simulink model "Tire1_basic02"  (R2022a)
settings: Solver=VariableStepAuto  StartTime=0.0  StopTime=100  RelTol=1e-3
undefined symbols (not defined in the file or in its folder): Mass
libraries: nesl_utility x2, fl_lib x1, sdl_lib x1
settings Model: Creator=amyyang  LastModifiedBy=amyyang
settings SolverCC: AlgebraicLoopSolver=TrustRegion
settings DebuggingCC: UnconnectedInputMsg=warning  UnconnectedOutputMsg=warning  UnconnectedLineMsg=warning  SFMachineParentedDataDiag=warning
settings RTWCC: DLArmComputeVersion=19.05
settings SimscapeCC: SimscapeLogType=local  SimscapeLogToSDI=on  SimscapeLogLimitData=off

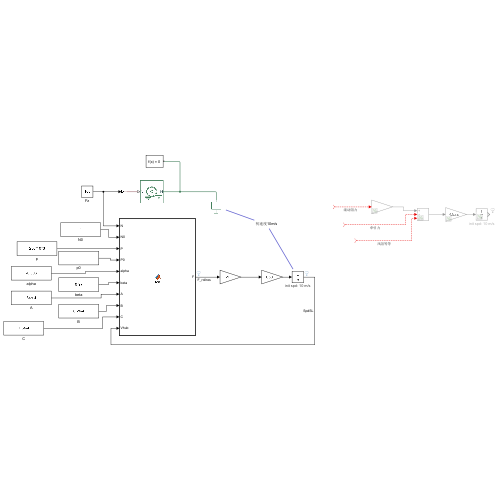
[thumbnail: Simulink's stored preview of the top-level diagram]
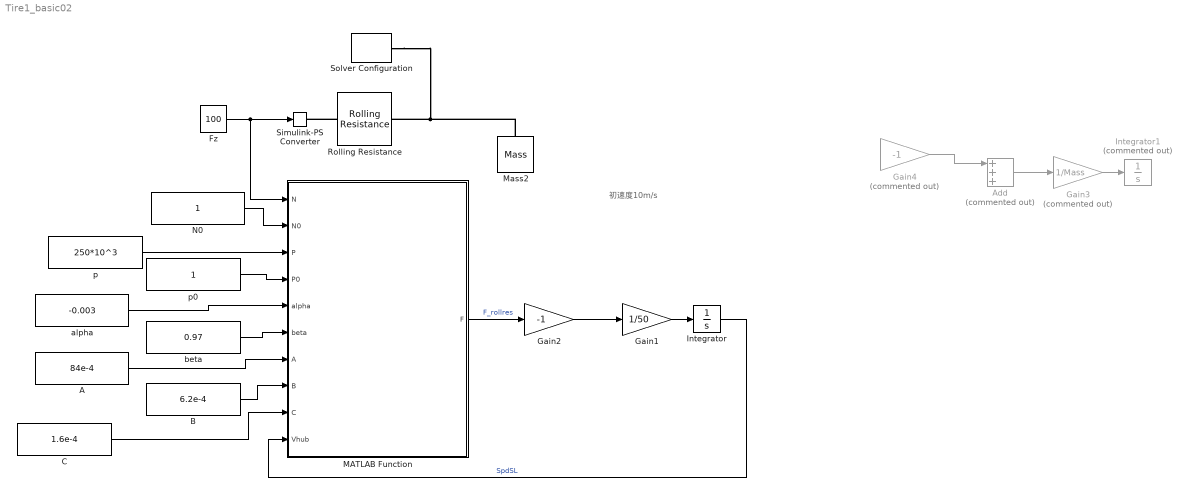
== system Tire1_basic02 ==
  note: 初速度10m/s
  A : Constant  Value=84e-4
  Add : Sum  Commented=on  Inputs=+++
  B : Constant  Value=6.2e-4
  C : Constant  Value=1.6e-4
  Fz : Constant  Value=100
  Gain1 : Gain  Gain=1/50
  Gain2 : Gain  Gain=-1
  Gain3 : Gain  Commented=on  Gain=1/Mass
  Gain4 : Gain  Commented=on  Gain=-1
  Integrator : Integrator  InitialCondition=10
      settings: AttributesFormatString=init spd: %<InitialCondition> m/s
  Integrator1 : Integrator  Commented=on  InitialCondition=10
      settings: AttributesFormatString=init spd: %<InitialCondition> m/s
  MATLAB Function : MATLAB Function  TreatAsAtomicUnit=on
  Mass2 : fl_lib/Mechanical/Translational Elements/Mass  mass=50 kg  num_ports=foundation.enum.numPorts2.one  v_specify=on  v_priority=High  v=10 m/s  v_nominal_specify=off  v_nominal_unit=m/s  v_nominal_value=1  f_specify=off  f_priority=None  f=0 N  f_nominal_specify=off  f_nominal_unit=N  f_nominal_value=1
      settings: SourceProductBaseCode=PW,SS,VE
  N0 : Constant
  Rolling Resistance : sdl_lib/Tires & Vehicles/Tire Subcomponents/Rolling Resistance  model=2  coeff=0.015  p_tire=250e3 Pa  alpha=-0.003  beta=0.97  coeff_a=84e-4  coeff_b=6.2e-4 s/m  coeff_c=1.6e-4 s^2/m^2  v_thr=0.001 m/s
      settings: SourceProductBaseCode=LD  LogSimulationData=on  InternalSimscapePortConfiguration="{\"Bottom\":[],\"Left\":[{\"id\":\"N\",\"label\":\"N\",\"type\":\"input\"}],\"Right\":[{\"id\":\"H\",\"label\":\"H\",\"type\":\"foundation.mechanical.translational.translational\"}],\"Top\":[]}"
  Simulink-PS Converter : nesl_utility/Simulink-PS Converter  PhysicalDomain=network_engine_domain  SubClassName=ps_input  LeftPortType=input  RightPortType=output  PseudoPeriodic=off  Frequencies=[]  NoiseDistribution=none  NoiseParameters=[]  Unit=N  AffineConversion=off  FilteringAndDerivatives=provide  SimscapeFilterOrder=1  InputFilterTimeConstant=0.001  UdotUserProvided=0
      settings: SourceProductBaseCode=SS,PW,VE
  Solver Configuration : nesl_utility/Solver Configuration  PhysicalDomain=network_engine_domain  SubClassName=solver  LeftPortType=input  RightPortType=generic  Tones=[]  Harmonics=[]  SimulateNoise=off  Profile=off  UseLocalSampling=off  EnableSwitchedLinearOptims=on  FrequencyDomain=off  UseCCode=off  RelTol=0.001  AbsTol=1e-06  MinStep=1e-09  ToWorkspace=off  RevertToSquareIcSolve=off  NumHomotopyIterations=100  PhasorMode=off  PhasorModeNumHarmonics=1  IndexReductionMethod=DerivativeReplacement  DoDC=off  ResidualTolerance=1e-09  UseLocalSolver=off  LocalSolverChoice=NE_BACKWARD_EULER_ADVANCER  LocalSolverSampleTime=0.001  DoFixedCost=off  MaxNonlinIter=3  MaxModeIter=2  ComputeImpulses=off  ImpulseIterations=2  LinearAlgebra=auto  LinearAlgebraNumThread=0  EquationFormulation=NE_TIME_EF  DelaysMemoryBudget=1024  AutomaticFiltering=on  FilteringTimeConstant=0.001  PartitionStorageMethod=AS_NEEDED  PartitionMemoryBudget=1024  PartitionMethod=ROBUST
      settings: SourceProductBaseCode=SS,PW,VE
  alpha : Constant  Value=-0.003
  beta : Constant  Value=0.97
  p : Constant  Value=250*10^3
  p0 : Constant
  wires:
  Fz/1 -> MATLAB Function/1(N), Simulink-PS Converter/1
  p/1 -> MATLAB Function/3(P)
  p0/1 -> MATLAB Function/4(P0)
  alpha/1 -> MATLAB Function/5(alpha)
  beta/1 -> MATLAB Function/6(beta)
  B/1 -> MATLAB Function/8(B)
  C/1 -> MATLAB Function/9(C)
  A/1 -> MATLAB Function/7(A)
  Gain1/1 -> Integrator/1
  MATLAB Function/1(F) -> Gain2/1  "F_rollres"
  Integrator/1 -> MATLAB Function/10(Vhub)  "SpdSL"
  N0/1 -> MATLAB Function/2(N0)
  Gain2/1 -> Gain1/1
  Gain3/1 -> Integrator1/1
  Add/1 -> Gain3/1
  Gain4/1 -> Add/1
  ? -> Add/2  "牵引力"
  ? -> Gain4/1  "滚动阻力"
  ? -> Add/3  "风阻等等"
  connections:
  Rolling Resistance/LConn1 -- Simulink-PS Converter/RConn1
  Mass2/LConn1 -- Solver Configuration/RConn1 -- Rolling Resistance/RConn1

== matlab function Tire1_basic02/MATLAB Function ==
  data: N input; N0 input; P input; F output; P0 input; alpha input; beta input; A input; B input; C input; Vhub input
function F = fcn(N,N0,P,P0,alpha,beta,A,B,C,Vhub)

F = (P/P0)^alpha * (N/N0)^beta*(A + B*abs(Vhub) + C* Vhub^2);
